simulink model "gm_hdlcoder_led_blinking_4bit_interface"  (R2016a)
settings: Solver=FixedStepDiscrete  SolverMode=SingleTasking  StartTime=0.0  StopTime=250  RelTol=1e-3
InitFcn:
  | Ts = 1e-3;
libraries: alterasoclib x3, simulink x2
settings Model: Creator=wchen  LastModifiedBy=d57w762
settings SolverCC: PositivePriorityOrder=on
settings DataIOCC: LimitDataPoints=on  SaveFormat=Array  SaveOutput=off  SignalLogging=off  SaveTime=off
settings OptimizationCC: BlockReduction=off  ConditionallyExecuteInputs=off  ExpressionDepthLimit=2147483647  OptimizeModelRefInitCode=on  LifeSpan=1  MaxStackSize=64
settings DebuggingCC: AlgebraicLoopMsg=error  UnderspecifiedInitializationDetection=Classic  MergeDetectMultiDrivingBlocksExec=none  SolverPrmCheckMsg=warning  SingleTaskRateTransMsg=error  ParameterPrecisionLossMsg=none  StateNameClashWarn=warning
settings HardwareCC: ProdBitPerPointer=32  ProdLargestAtomicInteger=Long  ProdLargestAtomicFloat=Double  ProdWordSize=32  ProdHWDeviceType=ARM Compatible->ARM Cortex  TargetEndianess=LittleEndian
settings ModelReferenceCC: PropagateSignalLabelsOutOfModel=off
settings RTWCC: SystemTargetFile=ert.tlc  HardwareBoard=Altera Cyclone V SoC development kit  TemplateMakefile=ert_default_tmf  GenerateReport=on  Toolchain=ARM Development Studio Altera Edition (DS-5 AE)  IncludeHyperlinkInReport=on  LaunchReport=on  GenerateTraceInfo=on  GenerateTraceReport=on  GenerateTraceReportSl=on  GenerateTraceReportSf=on  GenerateTraceReportEml=on
settings CodeAppCC: ForceParamTrailComments=on  IgnoreCustomStorageClasses=off  OperatorAnnotations=on  SimulinkDataObjDesc=on  SFDataObjDesc=on  MATLABFcnDesc=on  InsertBlockDesc=on  MATLABSourceComments=on
settings ConfigComp: CovModelRefEnable=Off  CovSFcnEnable=off

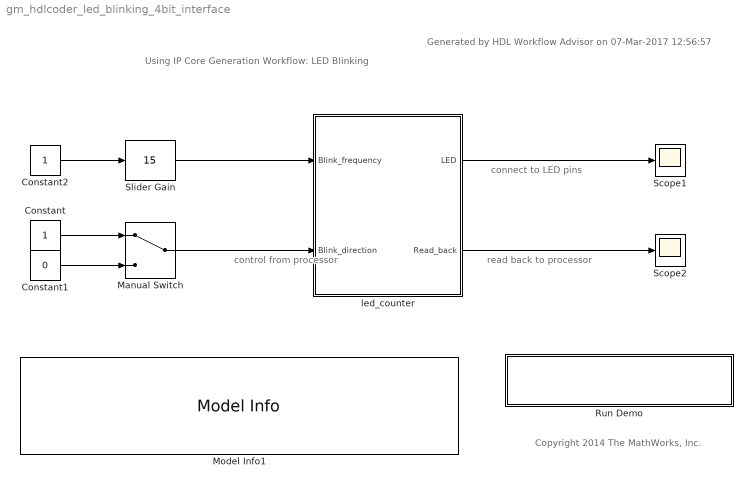
== system gm_hdlcoder_led_blinking_4bit_interface ==
  note: read back to
      | processor
  note: connect to
      | LED pins
  note: control from
      | processor
  note: Using IP Core Generation Workflow: LED Blinking
  note: Copyright 2014 The MathWorks, Inc.
  note: Generated by HDL Workflow Advisor on 07-Mar-2017 12:56:57
  Constant : Constant  OutDataTypeStr=boolean  SampleTime=Ts
  Constant1 : Constant  Value=0  OutDataTypeStr=boolean  SampleTime=Ts
  Constant2 : Constant  OutDataTypeStr=fixdt(0, 4, 0)  SampleTime=Ts
  Manual Switch : ManualSwitch
  Model Info1 : simulink/Model-Wide Utilities/Model Info  Frame=on  DisplayStringWithTags=|  HorizontalTextAlignment=Left  LeftAlignmentValue=0.02  SourceBlockDiagram=gm_hdlcoder_led_blinking_4bit_interface  TagMaxNumber=20
      | This example shows how to use HDL Workflow Advisor to    
      | generate a custom IP core which blink LEDs on FPGA board.
      |                                                          
      | In MATLAB, type the following:                           
      |   hdladvisor('hdlcoder_led_blinking_4bit/led_counter')
  Run Demo : Subsystem
      settings: OpenFcn=hdladvisor([bdroot, '/led_counter'])
      mask Display: disp('Launch HDL Workflow Advisor')
  Scope1 : Scope
  Scope2 : Scope
  Slider Gain : simulink/Math Operations/Slider Gain  low=0  gain=15  high=15
  led_counter : Subsystem  TreatAsAtomicUnit=on  mask(AXI4-Lite/AXI4 Interface){}
      mask help:
      | This is an automatically generated subsystem block.
      | This contains the AXI interface blocks that communicate with the led_count_ip IPCore generated from hdlcoder_led_blinking_4bit/led_counter subsystem.
      mask Display: disp(sprintf('Altera SoC \nAXI Interface'));
  wires:
  led_counter/1(LED) -> Scope1/1
  led_counter/2(Read_back) -> Scope2/1
  Slider Gain/1 -> led_counter/1(Blink_frequency)
  Constant2/1 -> Slider Gain/1
  Manual Switch/1 -> led_counter/2(Blink_direction)
  Constant1/1 -> Manual Switch/2
  Constant/1 -> Manual Switch/1

== system gm_hdlcoder_led_blinking_4bit_interface/Run Demo ==

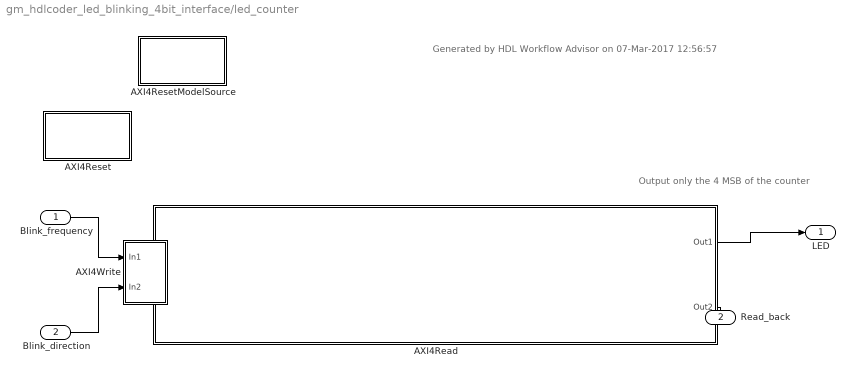
== system gm_hdlcoder_led_blinking_4bit_interface/led_counter ==
  note: Output only the 4 MSB of the counter
  note: Generated by HDL Workflow Advisor on 07-Mar-2017 12:56:57
  Blink_frequency : Inport  OutDataTypeStr=fixdt(0, 4, 0)
  Blink_direction : Inport  Port=2  OutDataTypeStr=boolean
  AXI4Read : Subsystem  Priority=10
  AXI4Reset : Subsystem  mask(System Initialize){ShowInLibBrowser=0}
      mask prompts: ShowInLibBrowser "Simulink:masks:CustCodeMaskParam1_MP"
      settings: CopyFcn=cccopyfcn(gcb)  OpenFcn=ccopenfcn('System Initialize Function')
      mask Help: eval('feval(''rtwprivate'',''rtwhelpview'',''rtw_sys_initialize_block'')');
      mask Display: disp('System\nInitialize');
  AXI4ResetModelSource : Subsystem  mask(Model Source){ShowInLibBrowser=0}
      mask prompts: ShowInLibBrowser "Simulink:masks:CustCodeMaskParam1_MP"
      settings: CopyFcn=cccopyfcn(gcb)  OpenFcn=ccopenfcn('Model Source')
      mask Help: eval('feval(''rtwprivate'',''rtwhelpview'',''rtw_model_source_block'')');
      mask Display: disp('Model\nSource');
  AXI4Write : Subsystem  Priority=1
  LED : Outport
  Read_back : Outport  Port=2
  wires:
  Blink_frequency/1 -> AXI4Write/1(In1)
  Blink_direction/1 -> AXI4Write/2(In2)
  AXI4Read/1(Out1) -> LED/1
  AXI4Read/2(Out2) -> Read_back/1

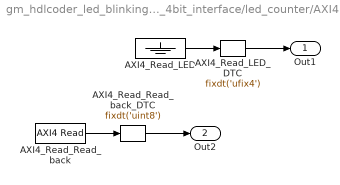
== system gm_hdlcoder_led_blinking_4bit_interface/led_counter/AXI4Read ==
  AXI4_Read_LED : Ground
  AXI4_Read_LED_DTC : DataTypeConversion  OutDataTypeStr=fixdt('ufix4')  ConvertRealWorld=Stored Integer (SI)
  AXI4_Read_Read_back : alterasoclib/AXI4 Read  Priority=3  DeviceName=/dev/mwipcore  RegisterOffset=hex2dec('108')  DataType=uint32  SampleTime=0.001  BlockPlatform=ALTERASOC
  AXI4_Read_Read_back_DTC : DataTypeConversion  OutDataTypeStr=fixdt('uint8')  ConvertRealWorld=Stored Integer (SI)
  Out1 : Outport
  Out2 : Outport  Port=2
  wires:
  AXI4_Read_LED/1 -> AXI4_Read_LED_DTC/1
  AXI4_Read_Read_back_DTC/1 -> Out2/1
  AXI4_Read_Read_back/1 -> AXI4_Read_Read_back_DTC/1
  AXI4_Read_LED_DTC/1 -> Out1/1

== system gm_hdlcoder_led_blinking_4bit_interface/led_counter/AXI4Reset ==

== system gm_hdlcoder_led_blinking_4bit_interface/led_counter/AXI4ResetModelSource ==

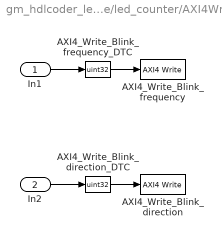
== system gm_hdlcoder_led_blinking_4bit_interface/led_counter/AXI4Write ==
  In1 : Inport
  In2 : Inport  Port=2
  AXI4_Write_Blink_direction : alterasoclib/AXI4 Write  Priority=2  DeviceName=/dev/mwipcore  RegisterOffset=hex2dec('104')  BlockPlatform=ALTERASOC
  AXI4_Write_Blink_direction_DTC : DataTypeConversion  OutDataTypeStr=uint32  ConvertRealWorld=Stored Integer (SI)
  AXI4_Write_Blink_frequency : alterasoclib/AXI4 Write  Priority=1  DeviceName=/dev/mwipcore  RegisterOffset=hex2dec('100')  BlockPlatform=ALTERASOC
  AXI4_Write_Blink_frequency_DTC : DataTypeConversion  OutDataTypeStr=uint32  ConvertRealWorld=Stored Integer (SI)
  wires:
  AXI4_Write_Blink_direction_DTC/1 -> AXI4_Write_Blink_direction/1
  In2/1 -> AXI4_Write_Blink_direction_DTC/1
  AXI4_Write_Blink_frequency_DTC/1 -> AXI4_Write_Blink_frequency/1
  In1/1 -> AXI4_Write_Blink_frequency_DTC/1
